simulink model "lateral_autopilot_2d"  (R2018b)
settings: Solver=VariableStepAuto  StartTime=0.0  StopTime=500  RelTol=1e-3
values from neighbouring files (symbols this model uses):
  a_phi_1 = 2.87    [lateral_autopilot_2e_params.m]
  a_phi_2 = -0.65    [lateral_autopilot_2e_params.m]
  d = 1.5    [lateral_autopilot_2e_params.m]
  g = 9.81    [lateral_autopilot_2e_params.m]
  kd_phi = (2*zeta_phi*omega_n_phi-a_phi_1)/a_phi_2    [lateral_autopilot_2e_params.m]
  ki_chi = omega_chi_phi^2*vg/g    [lateral_autopilot_2e_params.m]
  kp_chi = 2*zeta_chi*omega_chi_phi*vg/g    [lateral_autopilot_2e_params.m]
  kp_phi = (aileron_max/error_max)*sign(a_phi_2)    [lateral_autopilot_2e_params.m]
  vg = 580*km_h2m_s    (= 161.111111111)    [lateral_autopilot_2e_params.m]
libraries: simulink_extras x3, simulink x1
settings Model: Creator=dino  LastModifiedBy=dino

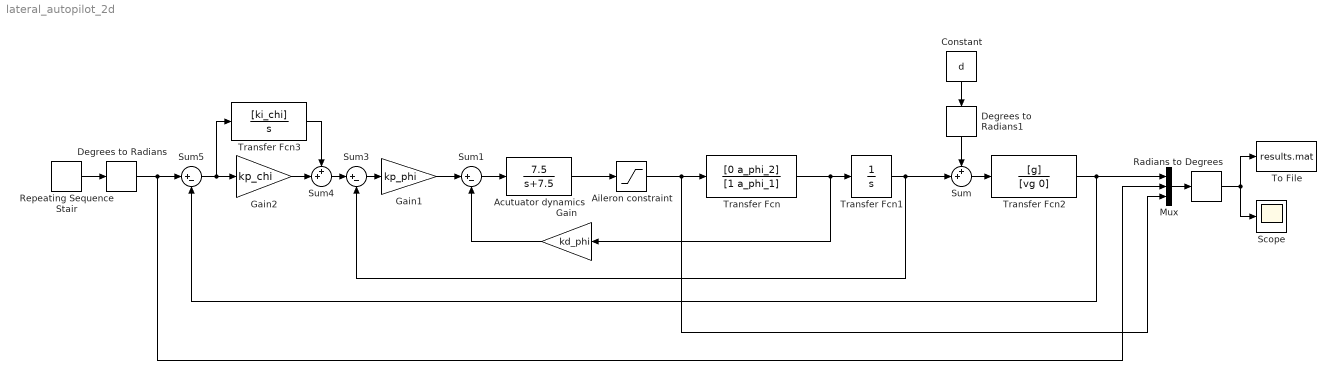
== system lateral_autopilot_2d ==
  Acutuator dynamics : TransferFcn  Numerator=[0 7.5]  Denominator=[1 7.5]
  "Aileron constraint " : Saturate  UpperLimit=30*deg2rad  LowerLimit=-30*deg2rad
  Constant : Constant  Value=d
  Degrees to Radians : simulink_extras/Transformations/Degrees to Radians
  Degrees to Radians1 : simulink_extras/Transformations/Degrees to Radians
  Gain : Gain  Gain=kd_phi
  Gain1 : Gain  Gain=kp_phi
  Gain2 : Gain  Gain=kp_chi
  Mux : Mux  Inputs=3
  Radians to Degrees : simulink_extras/Transformations/Radians to Degrees
  Repeating Sequence Stair : simulink/Sources/Repeating Sequence Stair  OutValues=step_series .'  tsamp=60  OutMin=[]  OutMax=[]  OutDataTypeStr=double  OutputDataTypeScalingMode=double  OutDataType=fixdt(0,8)  ConRadixGroup=Best Precision: Vector-wise  OutScaling=2^-12
  Scope : Scope
  Sum : Sum  Inputs=++|
  Sum1 : Sum  Inputs=|+-
  Sum3 : Sum  Inputs=|+-
  Sum4 : Sum  Inputs=++|
  Sum5 : Sum  Inputs=|+-
  To File : ToFile  Filename=results.mat
  Transfer Fcn : TransferFcn  Numerator=[0 a_phi_2]  Denominator=[1 a_phi_1]
  Transfer Fcn1 : TransferFcn  Denominator=[1 0]
  Transfer Fcn2 : TransferFcn  Numerator=[g]  Denominator=[vg 0]
  Transfer Fcn3 : TransferFcn  Numerator=[ki_chi]  Denominator=[1 0]
  wires:
  Transfer Fcn/1 -> Gain/1, Transfer Fcn1/1
  Transfer Fcn1/1 -> Sum/2, Sum3/2
  Sum/1 -> Transfer Fcn2/1
  Gain/1 -> Sum1/2
  Gain1/1 -> Sum1/1
  Sum3/1 -> Gain1/1
  Sum4/1 -> Sum3/1
  Gain2/1 -> Sum4/2
  Sum5/1 -> Transfer Fcn3/1, Gain2/1
  Transfer Fcn3/1 -> Sum4/1
  Repeating Sequence Stair/1 -> Degrees to Radians/1
  Mux/1 -> Radians to Degrees/1
  Degrees to Radians/1 -> Sum5/1, Mux/2
  Constant/1 -> Degrees to Radians1/1
  Degrees to Radians1/1 -> Sum/1
  Transfer Fcn2/1 -> Sum5/2, Mux/1
  Sum1/1 -> Acutuator dynamics/1
  Acutuator dynamics/1 -> "Aileron constraint "/1
  "Aileron constraint "/1 -> Mux/3, Transfer Fcn/1
  Radians to Degrees/1 -> Scope/1, To File/1
